simulink model "InductionMotor"  (R2019a)
settings: Solver=VariableStepAuto  StartTime=0.0  StopTime=2  RelTol=1e-3
libraries: powerlib x10, powerlib_meascontrol x2, BELBICtoolbox x1
settings Model: Creator=pavan  LastModifiedBy=pavan
settings SolverCC: AlgebraicLoopSolver=LineSearch

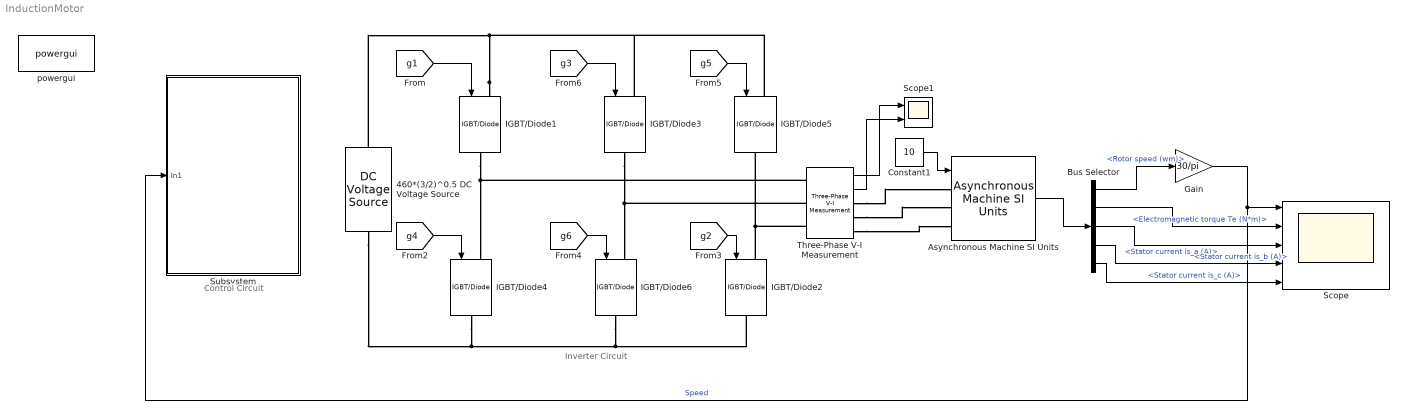
== system InductionMotor ==
  note: Control Circuit
  note: Inverter Circuit
  "460*(3/2)^0.5 DC Voltage Source " : powerlib/Electrical Sources/DC Voltage Source  Amplitude=400*(1.5)^0.5  Measurements=None
      settings: SourceProductName=Simscape Electrical
  Asynchronous Machine SI Units : powerlib/Machines/Asynchronous Machine SI Units  RotorType=Squirrel-cage  PresetModel="17:  20 HP (15KW)   400 V 50Hz 1460 RPM"  MechanicalLoad=Torque Tm  ShowDetailedParameters=on  ReferenceFrame=Rotor  Units=SI  MeasurementBus=off  NominalParameters=[1.5e+04 400 50]  Stator=[0.2147 0.000991]  Rotor=[0.2205 0.000991]  Cage1=[0.4155 0.002066]  Cage2=[0.4168 0.0003495]  Lm=0.06419  Mechanical=[0.102 0.009541 2]  PolePairs=2  InitialConditions=[0 0 0 0 0 0 0 0]  SimulateSaturation=off  Saturation=[14.03593122, 27.81365428, 53.79336849, 72.68890987, 97.98006896, 148.6815601, 215.7428561, 302.9841135, 428.7778367 ; 230, 322, 414, 460, 506, 552, 598, 644, 690]  LoadFlowParameters=1492000  TsPowergui=0  TsBlock=-1  IterativeModel=Trapezoidal non iterative  IterativeDiscreteModel=Trapezoidal non iterative  Pmec=1.492e+006
      settings: SourceProductName=Simscape Electrical
  Bus Selector : BusSelector  OutputSignals=Mechanical.Rotor speed (wm),Mechanical.Electromagnetic torque Te (N*m),Stator measurements.Stator current is_a (A),Stator measurements.Stator current is_b (A),Stator measurements.Stator current is_c (A)
  Constant1 : Constant  Value=10
  Gain : Gain  Gain=30/pi
  "IGBT/Diode1 " : powerlib/Power Electronics/IGBT//Diode  Ron=1e-3  Rs=1e5  Cs=inf  Measurements=off
      settings: SourceProductName=Simscape Electrical
  "IGBT/Diode2 " : powerlib/Power Electronics/IGBT//Diode  Ron=1e-3  Rs=1e5  Cs=inf  Measurements=off
      settings: SourceProductName=Simscape Electrical
  "IGBT/Diode3 " : powerlib/Power Electronics/IGBT//Diode  Ron=1e-3  Rs=1e5  Cs=inf  Measurements=off
      settings: SourceProductName=Simscape Electrical
  "IGBT/Diode4 " : powerlib/Power Electronics/IGBT//Diode  Ron=1e-3  Rs=1e5  Cs=inf  Measurements=off
      settings: SourceProductName=Simscape Electrical
  "IGBT/Diode5 " : powerlib/Power Electronics/IGBT//Diode  Ron=1e-3  Rs=1e5  Cs=inf  Measurements=off
      settings: SourceProductName=Simscape Electrical
  "IGBT/Diode6 " : powerlib/Power Electronics/IGBT//Diode  Ron=1e-3  Rs=1e5  Cs=inf  Measurements=off
      settings: SourceProductName=Simscape Electrical
  Scope : Scope  NumInputPorts=5
  Scope1 : Scope  NumInputPorts=2
  Subsystem : Subsystem
  Three-Phase V-I Measurement : powerlib/Measurements/Three-Phase V-I Measurement  VoltageMeasurement=phase-to-phase  SetLabelV=off  LabelV=Vabc  Vpu=off  VpuLL=off  CurrentMeasurement=yes  SetLabelI=off  LabelI=Iabc  Ipu=off  Pbase=100e6  Vbase=500e3  OutputType=Complex  PhasorSimulation=off  PSBequivalent=0
      settings: SourceProductName=Simscape Electrical
  powergui : powerlib/powergui  Priority=1  SimulationMode=Discrete  SampleTime=50e-6  frequency=60  Iterations=50  frequencyindice=50  Pbase=100e6  ErrMax=1e-4  UnitsV=kV  UnitsW=MW  buscounter=0  FunctionMessages=off  echomessages=off  EnableUseOfTLC=off  CurrentSourceSwitches=off  DisableSnubberDevices=off  DisableRonSwitches=off  DisableVfSwitches=off  DisplayEquations=off  AutomaticDiscreteSolvers=off  SolverType=Tustin/Backward Euler (TBE)  Interpol=off  ExternalGateDelay=off  methode=off  Ts=100  x0status=blocks  SPID=on  SwTol=0  HookPort=off  NonlinearTolerance=0  nMaxIteration=15  ContinueOnMaxIteration=off  RestoreLinks=warning  ResistiveCurrentMeasurement=off  Frange=[0:2:500]  Ylog=off  Xlog=on  ShowGrid=off  save=off  variable=ZData  structure=0  ZoomFFT=off  StartTime=0.0  cycles=1  DisplayStyle=1  fundamental=60  FreqAxis=off  MaxFrequency=1000  frequencyindicesteady=1  RmsSteady=1  display=off
      settings: SourceProductName=Simscape Electrical
  wires:
  Bus Selector/3 -> Scope/3  "<Stator current is_a (A)>"
  Bus Selector/2 -> Scope/2  "<Electromagnetic torque Te (N*m)>"
  Three-Phase V-I Measurement/1 -> Scope1/1
  Three-Phase V-I Measurement/2 -> Scope1/2
  Bus Selector/1 -> Gain/1  "<Rotor speed (wm)>"
  Asynchronous Machine SI Units/1 -> Bus Selector/1
  Gain/1 -> Scope/1, Subsystem/1(In1)  "Speed"
  [g4] -> "IGBT/Diode4 "/1
  [g3] -> "IGBT/Diode3 "/1
  [g5] -> "IGBT/Diode5 "/1
  [g6] -> "IGBT/Diode6 "/1
  [g2] -> "IGBT/Diode2 "/1
  Bus Selector/5 -> Scope/5  "<Stator current is_c (A)>"
  [g1] -> "IGBT/Diode1 "/1
  Constant1/1 -> Asynchronous Machine SI Units/1
  Bus Selector/4 -> Scope/4  "<Stator current is_b (A)>"
  connections:
  "IGBT/Diode1 "/LConn1 -- "IGBT/Diode5 "/LConn1 -- "IGBT/Diode3 "/LConn1 -- "460*(3/2)^0.5 DC Voltage Source "/RConn1
  "IGBT/Diode4 "/RConn1 -- "460*(3/2)^0.5 DC Voltage Source "/LConn1 -- "IGBT/Diode2 "/RConn1 -- "IGBT/Diode6 "/RConn1
  "IGBT/Diode2 "/LConn1 -- "IGBT/Diode5 "/RConn1 -- Three-Phase V-I Measurement/LConn3
  "IGBT/Diode1 "/RConn1 -- "IGBT/Diode4 "/LConn1 -- Three-Phase V-I Measurement/LConn1
  "IGBT/Diode3 "/RConn1 -- Three-Phase V-I Measurement/LConn2 -- "IGBT/Diode6 "/LConn1
  Three-Phase V-I Measurement/RConn1 -- Asynchronous Machine SI Units/LConn1
  Three-Phase V-I Measurement/RConn2 -- Asynchronous Machine SI Units/LConn2
  Three-Phase V-I Measurement/RConn3 -- Asynchronous Machine SI Units/LConn3

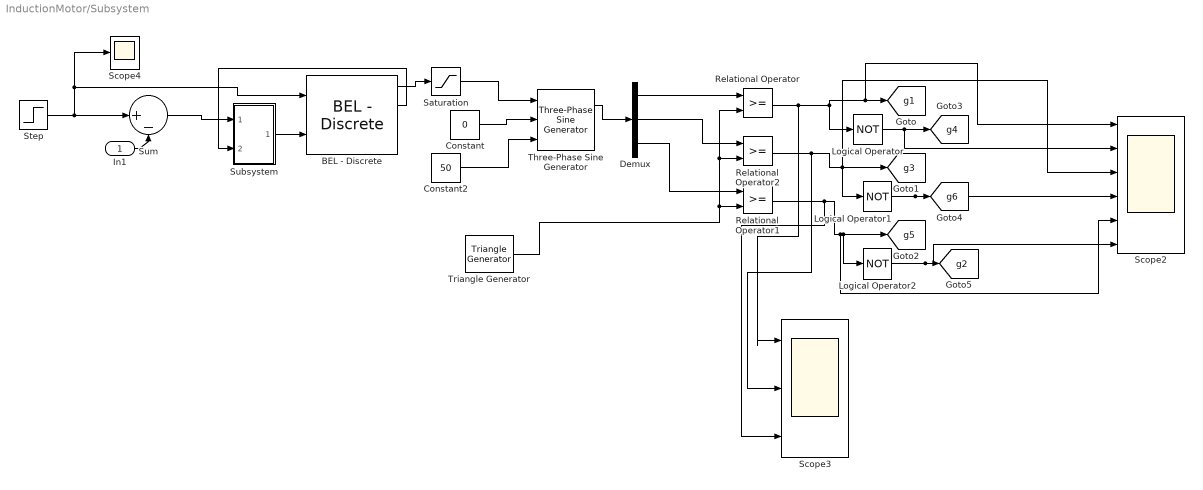
== system InductionMotor/Subsystem ==
  In1 : Inport
  BEL - Discrete : BELBICtoolbox/Discrete-time/BEL - Discrete  alfa=0.1  beta=0.06  V=25  Vth=30  W=0.1  T=1
      settings: SourceProductName=BELBIC Toolbox
  Constant : Constant  Value=0
  Constant2 : Constant  Value=50
  Demux : Demux  Outputs=3
  Logical Operator : Logic  Operator=NOT  IconShape=distinctive  AllPortsSameDT=off  OutDataTypeStr=boolean
  Logical Operator1 : Logic  Operator=NOT  IconShape=distinctive  AllPortsSameDT=off  OutDataTypeStr=boolean
  Logical Operator2 : Logic  Operator=NOT  IconShape=distinctive  AllPortsSameDT=off  OutDataTypeStr=boolean
  Relational Operator : RelationalOperator  OutDataTypeStr=boolean  RndMeth=Simplest
  Relational Operator1 : RelationalOperator  OutDataTypeStr=boolean  RndMeth=Simplest
  Relational Operator2 : RelationalOperator  OutDataTypeStr=boolean  RndMeth=Simplest
  Saturation : Saturate  UpperLimit=1  LowerLimit=-1
  Scope2 : Scope  NumInputPorts=6
  Scope3 : Scope  NumInputPorts=3
  Scope4 : Scope
  Step : Step  After=1460  SampleTime=0
  Subsystem : Subsystem
  Sum : Sum  Inputs=|+-
  Three-Phase Sine Generator : powerlib_meascontrol/Pulse & Signal Generators/Three-Phase Sine Generator  Ts=0
      settings: SourceProductName=Simscape Electrical  SourceProductBaseCode=PS
  Triangle Generator : powerlib_meascontrol/Pulse & Signal Generators/Triangle Generator  Freq=50  Phase=90  Ts=0
      settings: SourceProductName=Simscape Electrical
  tag scope: g1=global, g2=global, g3=global, g4=global, g5=global, g6=global
  wires:
  Relational Operator/1 -> Scope3/1, Logical Operator/1, Scope2/1, [g1]
  Logical Operator2/1 -> Scope2/6, [g2]
  Relational Operator1/1 -> Scope3/3, [g5], Logical Operator2/1, Scope2/5
  Relational Operator2/1 -> Scope3/2, [g3], Scope2/3, Logical Operator1/1
  Demux/2 -> Relational Operator2/1
  Three-Phase Sine Generator/1 -> Demux/1
  Logical Operator1/1 -> Scope2/4, [g6]
  Demux/3 -> Relational Operator1/1
  Constant/1 -> Three-Phase Sine Generator/2
  Step/1 -> BEL - Discrete/1, Scope4/1, Sum/1
  Triangle Generator/1 -> Relational Operator1/2, Relational Operator2/2, Relational Operator/2
  Logical Operator/1 -> Scope2/2, [g4]
  Demux/1 -> Relational Operator/1
  In1/1 -> Sum/2
  Constant2/1 -> Three-Phase Sine Generator/3
  Subsystem/1(Out1) -> BEL - Discrete/2
  Sum/1 -> Subsystem/1(In1)
  BEL - Discrete/1 -> Saturation/1
  Saturation/1 -> Three-Phase Sine Generator/1
  BEL - Discrete/2 -> Subsystem/2(In2)

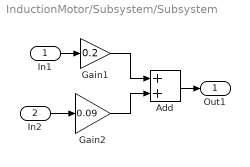
== system InductionMotor/Subsystem/Subsystem ==
  In1 : Inport
  In2 : Inport  Port=2
  Add : Sum
  Gain1 : Gain  Gain=0.2
  Gain2 : Gain  Gain=0.09
  Out1 : Outport
  wires:
  In1/1 -> Gain1/1
  Gain2/1 -> Add/2
  In2/1 -> Gain2/1
  Add/1 -> Out1/1
  Gain1/1 -> Add/1
